simulink model "OS_Inverse_Dynamics_Control"  (R2023b)
settings: Solver=ode1  StartTime=0.0  StopTime=50  FixedStep=Tc  RelTol=1e-5
values from neighbouring files (symbols this model uses):
  Tc = 0.001    [scara_parameters.m]
undefined symbols (not defined in the file or in its folder): DiscIntNeverNeededParam, K_D_os_invdyn, K_I_os_invdyn, K_P_os_invdyn, mload, q0
settings Model: Creator=emman  LastModifiedBy=emman

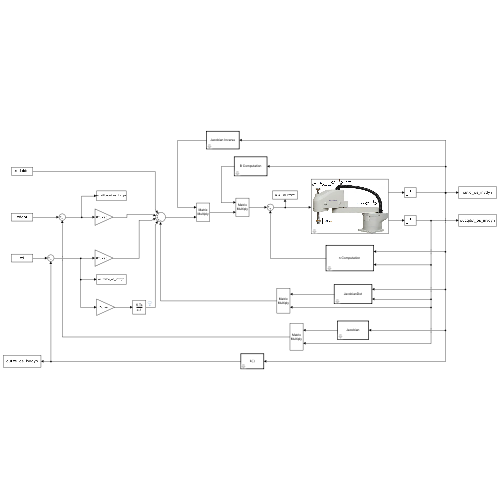
[thumbnail: Simulink's stored preview of the top-level diagram]
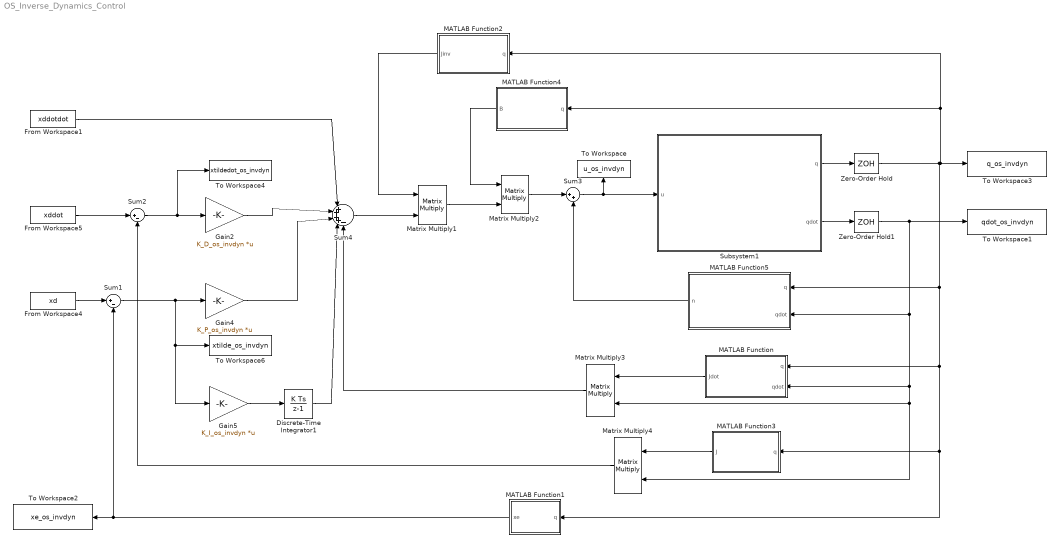
== system OS_Inverse_Dynamics_Control ==
  Discrete-Time Integrator1 : DiscreteIntegrator  InitialCondition=[0 0 0 0]'  SampleTime=Tc  ICPrevOutput=DiscIntNeverNeededParam  ICPrevScaledInput=DiscIntNeverNeededParam
  From Workspace1 : FromWorkspace  VariableName=xddotdot  SampleTime=Tc
  From Workspace4 : FromWorkspace  VariableName=xd  SampleTime=Tc
  From Workspace5 : FromWorkspace  VariableName=xddot  SampleTime=Tc
  Gain2 : Gain  Gain=K_D_os_invdyn  Multiplication=Matrix(K*u) (u vector)
  Gain4 : Gain  Gain=K_P_os_invdyn  Multiplication=Matrix(K*u) (u vector)
  Gain5 : Gain  Gain=K_I_os_invdyn  Multiplication=Matrix(K*u) (u vector)
  MATLAB Function : MATLAB Function  TreatAsAtomicUnit=on
  MATLAB Function1 : MATLAB Function  TreatAsAtomicUnit=on
  MATLAB Function2 : MATLAB Function  TreatAsAtomicUnit=on
  MATLAB Function3 : MATLAB Function  TreatAsAtomicUnit=on
  MATLAB Function4 : MATLAB Function  TreatAsAtomicUnit=on
  MATLAB Function5 : MATLAB Function  TreatAsAtomicUnit=on
  Matrix Multiply{1..4} (4 alike) : Product  Multiplication=Matrix(*)
  Subsystem1 : Subsystem
      mask Display: image('SCARA.png');
  Sum1 : Sum  Inputs=|+-
  Sum2 : Sum  Inputs=|+-
  Sum3 : Sum  Inputs=|++
  Sum4 : Sum  Inputs=|++++-
  To Workspace : ToWorkspace  VariableName=u_os_invdyn  SaveFormat=Structure With Time  SampleTime=-1
  To Workspace1 : ToWorkspace  VariableName=qdot_os_invdyn  SaveFormat=Structure With Time  SampleTime=-1
  To Workspace2 : ToWorkspace  VariableName=xe_os_invdyn  SaveFormat=Structure With Time  SampleTime=-1
  To Workspace3 : ToWorkspace  VariableName=q_os_invdyn  SaveFormat=Structure With Time  SampleTime=-1
  To Workspace4 : ToWorkspace  VariableName=xtildedot_os_invdyn  SaveFormat=Structure With Time  SampleTime=-1
  To Workspace6 : ToWorkspace  VariableName=xtilde_os_invdyn  SaveFormat=Structure With Time  SampleTime=-1
  Zero-Order Hold : ZeroOrderHold  SampleTime=Tc
  Zero-Order Hold1 : ZeroOrderHold  SampleTime=Tc
  wires:
  From Workspace4/1 -> Sum1/1
  Sum1/1 -> Gain4/1, Gain5/1, To Workspace6/1
  From Workspace5/1 -> Sum2/1
  Sum2/1 -> To Workspace4/1, Gain2/1
  Zero-Order Hold/1 -> MATLAB Function2/1(q), MATLAB Function4/1(q), To Workspace3/1, MATLAB Function1/1(q), MATLAB Function3/1(q), MATLAB Function/1(q), MATLAB Function5/1(q)
  From Workspace1/1 -> Sum4/1
  Gain2/1 -> Sum4/2
  Zero-Order Hold1/1 -> To Workspace1/1, MATLAB Function5/2(qdot), MATLAB Function/2(qdot), Matrix Multiply4/2, Matrix Multiply3/2
  Sum3/1 -> Subsystem1/1(u), To Workspace/1
  Subsystem1/1(q) -> Zero-Order Hold/1
  Subsystem1/2(qdot) -> Zero-Order Hold1/1
  Gain4/1 -> Sum4/3
  MATLAB Function1/1(xe) -> To Workspace2/1, Sum1/2
  MATLAB Function2/1(Jinv) -> Matrix Multiply1/1
  Sum4/1 -> Matrix Multiply1/2
  Matrix Multiply1/1 -> Matrix Multiply2/2
  MATLAB Function4/1(B) -> Matrix Multiply2/1
  MATLAB Function5/1(n) -> Sum3/2
  Matrix Multiply2/1 -> Sum3/1
  MATLAB Function/1(Jdot) -> Matrix Multiply3/1
  MATLAB Function3/1(J) -> Matrix Multiply4/1
  Matrix Multiply4/1 -> Sum2/2
  Gain5/1 -> Discrete-Time Integrator1/1
  Discrete-Time Integrator1/1 -> Sum4/4
  Matrix Multiply3/1 -> Sum4/5

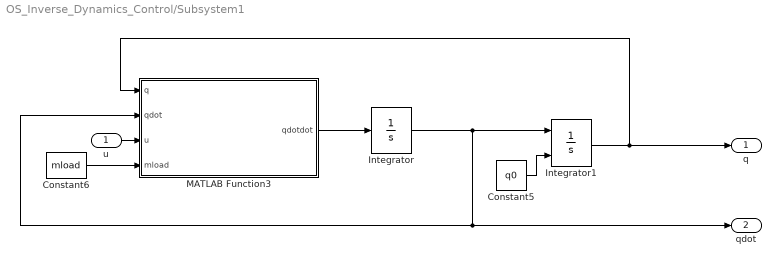
== system OS_Inverse_Dynamics_Control/Subsystem1 ==
  u : Inport
  Constant5 : Constant  Value=q0
  Constant6 : Constant  Value=mload
  Integrator : Integrator  InitialCondition=[0 0 0 0]'
  Integrator1 : Integrator  InitialConditionSource=external
  MATLAB Function3 : MATLAB Function  TreatAsAtomicUnit=on
  q : Outport
  qdot : Outport  Port=2
  wires:
  Constant6/1 -> MATLAB Function3/4(mload)
  Integrator/1 -> Integrator1/1, qdot/1, MATLAB Function3/2(qdot)
  u/1 -> MATLAB Function3/3(u)
  Integrator1/1 -> q/1, MATLAB Function3/1(q)
  MATLAB Function3/1(qdotdot) -> Integrator/1
  Constant5/1 -> Integrator1/2

== matlab function OS_Inverse_Dynamics_Control/Subsystem1/MATLAB Function3 ==
  data: q input; qdotdot output; qdot input; u input; mload input
function qdotdot = DirectDynamic(q,qdot,u,mload)
    
    %m
    a1 = 0.5;
    a2 = 0.5;
    l1 = 0.25;
    l2 = 0.25;
    
    %kg
    ml1 = 20;
    ml2 = 20;
    ml3 = 10;
    
    %rad/m
    kr1 = 1;
    kr2 = 1;
    kr3 = 50;
    kr4 = 20;
        
    %N*m*s/rad
    Fm1 = 0.00005;
    Fm2 = 0.00005;
    Fm3 = 0.01;
    Fm4 = 0.005;
    
    B = BComputation(q);

    %Christoffel Symbols
    c = zeros(4,4,4);
    
    %c_ijk = 1/2*(db_ij/dq_k + db_ik/dq_j - db_jk/dq_i)
    %For Example: c_112 = 1/2*(db_11/dq_2 + db_12/dq_1 - db_12/dq_1) =
    % = 1/2 * db_11/dq_2
    %Christoffel Symbols Properties:
    %c_iii = 0 since db_ii/dq_i = 0 for all i
    %c_ijk = c_ikj
    %Additionally b_ji = b_ij

    %Using the file InertiaMatrix.m in this folder it is possible to
    %visualize the matrix B(4x4) and the various b_11, b_12, b_21 and b_22
    %with the command (B(1,1), B(1,2), B(2,1) and B(2,2))

    c(1,1,2) = 1/2*(-2*a1*a2*ml3*sin(q(2))-2*a1*l2*ml2*sin(q(2)) + 0 ); 
    c(1,2,1) = c(1,1,2);
    
    %c_211 = 1/2*(db_21/dq_1 + db_21/dq_1 - db_11/dq_2) = -1/2 * db_11/dq_2
    %So c_211 = -c_112
    c(2,1,1) = -c(1,1,2);

    %c_122 = 1/2*(db_12/dq_2 + db_12/dq_2 - b_22/dq_1) = db_12/dq_2
    c(1,2,2) = -a1*a2*ml3*sin(q(2)) - a1*l2*ml2*sin(q(2));
    %It is possible to note that also c(1,2,2) = c(1,1,2)

    %c_212 = c_221 = 1/2*(db_21/dq_2 + db_22/dq_1 - db_12/dq_2) = 0
    %The other Christoffel Symbols are all nulls because B does not depend
    %on q(3) and q(4)
    C=zeros(4,4);

    %c(q,qdot)=C(q,qdot)*qdot
    %c_ik = c_ijk(q)qdot_j
    %c_ik is the ik element of the matrix C

    for i=1:4
        for j=1:4
            for k=1:4
                C(i,k)= C(i,k)+c(i,j,k)*qdot(j);    %C(i,k) in the second term is superfluous
            end
        end
    end
    
    %Gravity of link 3 (ml3) and load (mload)
    g = [0 0 9.81*(ml3+mload) 0]';

    %Viscous Friction
    Fv=diag([kr1^2*Fm1 kr2^2*Fm2 kr3^2*Fm3 kr4^2*Fm4]);

    %Acceleration
    qdotdot = inv(B)*(u-C*qdot-Fv*qdot-g);

end

== matlab function OS_Inverse_Dynamics_Control/MATLAB Function2 ==
  data: Jinv output; q input
function Jinv = JacobianInverse(q)

J = jacobian(q);

Jinv = inv(J);

end

== matlab function OS_Inverse_Dynamics_Control/MATLAB Function3 ==
  data: q input; J output
function J = Jac(q)
    
    J = jacobian(q);

end

== matlab function OS_Inverse_Dynamics_Control/MATLAB Function1 ==
  data: q input; xe output
function xe = DirKin(q)

    xe = k(q);

end

== matlab function OS_Inverse_Dynamics_Control/MATLAB Function ==
  data: q input; Jdot output; qdot input
function Jdot = JacobianDot(q,qdot)

    a1 = 0.5;
    a2 = 0.5;

    Jdot = [-a2*(qdot(1)+qdot(2))*cos(q(1)+q(2))-a1*qdot(1)*cos(q(1)) -a2*(qdot(1)+qdot(2))*cos(q(1)+q(2)) 0 0;
            -a2*(qdot(1)+qdot(2))*sin(q(1)+q(2))-a1*qdot(1)*sin(q(1)) -a2*(qdot(1)+qdot(2))*sin(q(1)+q(2)) 0 0;
            0 0 0 0;
            0 0 0 0];

end

== matlab function OS_Inverse_Dynamics_Control/MATLAB Function4 ==
  data: q input; B output
function B = BComputationOS_Inv_Dyn(q)
      
    B = BComputation(q);
    
end

== matlab function OS_Inverse_Dynamics_Control/MATLAB Function5 ==
  data: q input; n output; qdot input
function n = nComputation(q,qdot)
    
    %m
    a1 = 0.5;
    a2 = 0.5;
    
    %m
    l1 = 0.25;
    l2 = 0.25;
    
    %kg
    ml1 = 20;
    ml2 = 20;
    ml3 = 10;
    
    %rad/m
    kr1 = 1;
    kr2 = 1;
    kr3 = 50;
    kr4 = 20;
    
    
    %N*m*s/rad
    Fm1 = 0.00005;
    Fm2 = 0.00005;
    Fm3 = 0.01;
    Fm4 = 0.005;
    
    %NON-Linear Terms

    %Christoffel Symbols
    c = zeros(4,4,4);
    
    %c_ijk = 1/2*(db_ij/dq_k + db_ik/dq_j - db_jk/dq_i)
    %For Example: c_112 = 1/2*(db_11/dq_2 + db_12/dq_1 - db_12/dq_1) =
    % = 1/2 * db_11/dq_2
    %Christoffel Symbols Properties:
    %c_iii = 0 since db_ii/dq_i = 0 for all i
    %c_ijk = c_ikj
    %Additionally b_ji = b_ij

    %Using the file InertiaMatrix.m in this folder it is possible to
    %visualize the matrix B(4x4) and the various b_11, b_12, b_21 and b_22
    %with the command (B(1,1), B(1,2), B(2,1) and B(2,2))

    c(1,1,2) = 1/2*(-2*a1*a2*ml3*sin(q(2))-2*a1*l2*ml2*sin(q(2)) + 0 ); 
    c(1,2,1) = c(1,1,2);
    
    %c_211 = 1/2*(db_21/dq_1 + db_21/dq_1 - db_11/dq_2) = -1/2 * db_11/dq_2
    %So c_211 = -c_112
    c(2,1,1) = -c(1,1,2);

    %c_122 = 1/2*(db_12/dq_2 + db_12/dq_2 - b_22/dq_1) = db_12/dq_2
    c(1,2,2) = -a1*a2*ml3*sin(q(2)) - a1*l2*ml2*sin(q(2));
    %It is possible to note that also c(1,2,2) = c(1,1,2)

    %c_212 = c_221 = 1/2*(db_21/dq_2 + db_22/dq_1 - db_12/dq_2) = 0
    %The other Christoffel Symbols are all nulls because B does not depend
    %on q(3) and q(4)
    C=zeros(4,4);

    %c(q,qdot)=C(q,qdot)*qdot
    %c_ik = c_ijk(q)qdot_j
    %c_ik is the ik element of the matrix C

    for i=1:4
        for j=1:4
            for k=1:4
                C(i,k)= C(i,k)+c(i,j,k)*qdot(j);    %C(i,k) in the second term is superfluous
            end
        end
    end

    %Gravitational Term
    g = [0 0 ml3*9.81 0]';

    %Vicous Friction Term
    %To convert from the motor side to the joint side,
    % it is necessary to multiply by the transmission ratio.
    Fv = diag([kr1^2*Fm1 kr2^2*Fm2 kr3^2*Fm3 kr4^2*Fm4]);

    n = C*qdot + Fv*qdot + g;
end
